simulink model "control"  (R2017b)
settings: Solver=ode45  StartTime=0.0  StopTime=2  RelTol=1e-3
values from neighbouring files (symbols this model uses):
  duracion = in(9)    [GTCL_R3GDL.m]
  Kd = [1.3735e+01 2.5872e+01 0.2837e+01]    [Control.m]    (also in dsgn_PD.m = Kp.*Td)
  Ki = [0 0 0]    [Control.m]    (also in dsgn_PD.m = Kp./Ti)
  Kp = [7.4989e+02 1.4125e+03 1.5488e+02]    [Control.m]    (also in dsgn_PD.m = [2.1312e+06 8.4844e+05 4.5042e+05])
  n = in(7)    [GTCL_R3GDL.m]
  XYZfin = [in(4) in(5) in(6)]'    [GTCL_R3GDL.m]
undefined symbols (not defined in the file or in its folder): t_ini, XYZini
settings Model: Creator=fevaf  LastModifiedBy=Raúl

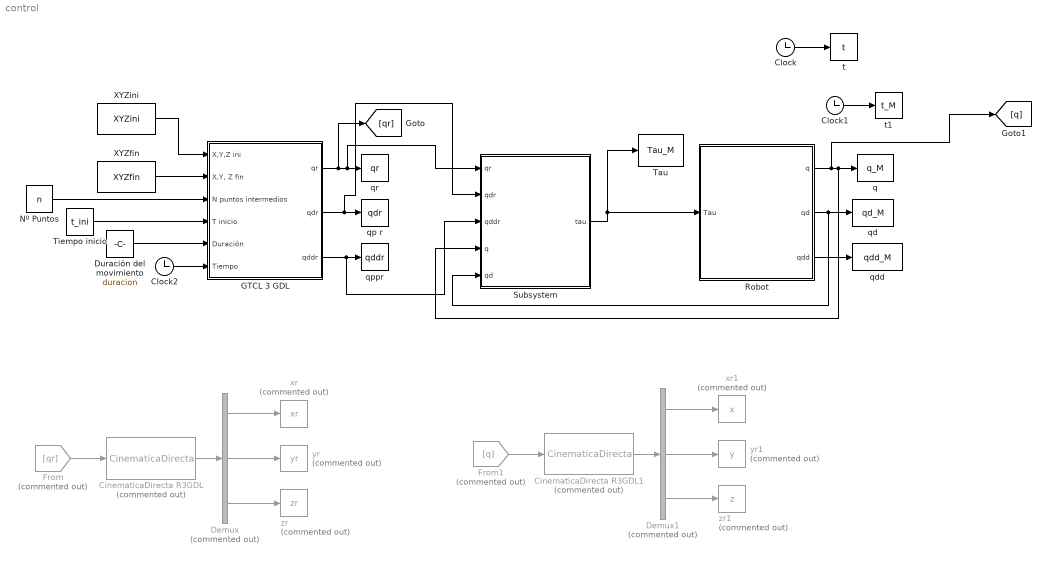
== system control ==
  CinematicaDirecta R3GDL : MATLABFcn  Commented=on  MATLABFcn=CinematicaDirecta
  CinematicaDirecta R3GDL1 : MATLABFcn  Commented=on  MATLABFcn=CinematicaDirecta
  Clock : Clock
  Clock1 : Clock
  Clock2 : Clock
  Demux : Demux  Commented=on  Outputs=3
  Demux1 : Demux  Commented=on  Outputs=3
  Duración del movimiento : Constant  Value=duracion
  From : From  Commented=on  GotoTag=qr
      settings: CloseFcn=tagdialog Close
  From1 : From  Commented=on  GotoTag=q
      settings: CloseFcn=tagdialog Close
  GTCL 3 GDL : Subsystem
  Nº Puntos : Constant  Value=n
  Robot : Subsystem
  Subsystem : Subsystem
  "Tau " : ToWorkspace  VariableName=Tau_M  SampleTime=-1
  Tiempo inicio : Constant  Value=t_ini
  XYZfin : Constant  Value=XYZfin
  XYZini : Constant  Value=XYZini
  q : ToWorkspace  VariableName=q_M  SampleTime=-1
  qd : ToWorkspace  VariableName=qd_M  SampleTime=-1
  qdd : ToWorkspace  VariableName=qdd_M  SampleTime=-1
  qp r : ToWorkspace  VariableName=qdr  SampleTime=-1
  qppr : ToWorkspace  VariableName=qddr  SampleTime=-1
  qr : ToWorkspace  VariableName=qr  SampleTime=-1
  t : ToWorkspace  VariableName=t  SampleTime=-1
  t1 : ToWorkspace  VariableName=t_M  SampleTime=-1
  xr : ToWorkspace  Commented=on  VariableName=xr  SampleTime=-1
  xr1 : ToWorkspace  Commented=on  VariableName=x  SampleTime=-1
  yr : ToWorkspace  Commented=on  VariableName=yr  SampleTime=-1
  yr1 : ToWorkspace  Commented=on  VariableName=y  SampleTime=-1
  zr : ToWorkspace  Commented=on  VariableName=zr  SampleTime=-1
  zr1 : ToWorkspace  Commented=on  VariableName=z  SampleTime=-1
  wires:
  Demux/3 -> zr/1
  Demux/1 -> xr/1
  Demux/2 -> yr/1
  XYZfin/1 -> GTCL 3 GDL/2("X,Y, Z fin")
  XYZini/1 -> GTCL 3 GDL/1(X,Y,Z ini)
  Tiempo inicio/1 -> GTCL 3 GDL/4(T inicio)
  GTCL 3 GDL/3(qddr) -> Subsystem/3(qddr), qppr/1
  CinematicaDirecta R3GDL/1 -> Demux/1
  GTCL 3 GDL/1(qr) -> Subsystem/1(qr), qr/1, [qr]
  Clock2/1 -> GTCL 3 GDL/6(Tiempo)
  Duración del movimiento/1 -> GTCL 3 GDL/5(Duración)
  From/1 -> CinematicaDirecta R3GDL/1
  GTCL 3 GDL/2(qdr) -> Subsystem/2(qdr), qp r/1
  Nº Puntos/1 -> GTCL 3 GDL/3(N puntos intermedios)
  Clock/1 -> t/1
  Subsystem/1("tau ") -> Robot/1(Tau), "Tau "/1
  Robot/2(qd) -> Subsystem/5(qd), qd/1
  Robot/1(q) -> [q], Subsystem/4(q), q/1
  Robot/3(qdd) -> qdd/1
  Clock1/1 -> t1/1
  From1/1 -> CinematicaDirecta R3GDL1/1
  Demux1/2 -> yr1/1
  CinematicaDirecta R3GDL1/1 -> Demux1/1
  Demux1/3 -> zr1/1
  Demux1/1 -> xr1/1

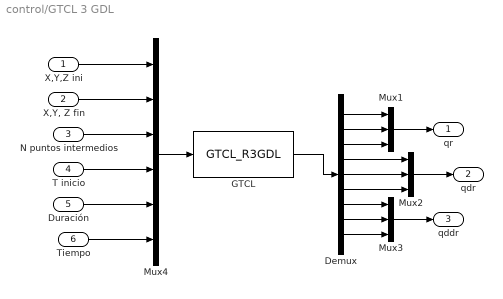
== system control/GTCL 3 GDL ==
  X,Y,Z ini : Inport
  "X,Y, Z fin" : Inport  Port=2
  N puntos intermedios : Inport  Port=3
  T inicio : Inport  Port=4
  Duración : Inport  Port=5
  Tiempo : Inport  Port=6
  Demux : Demux  Outputs=9
  GTCL : MATLABFcn  MATLABFcn=GTCL_R3GDL  OutputDimensions=9
  Mux1 : Mux  Inputs=3
  Mux2 : Mux  Inputs=3
  Mux3 : Mux  Inputs=3
  Mux4 : Mux  Inputs=6
  qr : Outport
  qdr : Outport  Port=2
  qddr : Outport  Port=3
  wires:
  Mux1/1 -> qr/1
  Mux4/1 -> GTCL/1
  X,Y,Z ini/1 -> Mux4/1
  "X,Y, Z fin"/1 -> Mux4/2
  N puntos intermedios/1 -> Mux4/3
  T inicio/1 -> Mux4/4
  Duración/1 -> Mux4/5
  Tiempo/1 -> Mux4/6
  GTCL/1 -> Demux/1
  Demux/1 -> Mux1/1
  Demux/2 -> Mux1/2
  Demux/3 -> Mux1/3
  Mux2/1 -> qdr/1
  Demux/4 -> Mux2/1
  Demux/5 -> Mux2/2
  Demux/6 -> Mux2/3
  Mux3/1 -> qddr/1
  Demux/7 -> Mux3/1
  Demux/8 -> Mux3/2
  Demux/9 -> Mux3/3

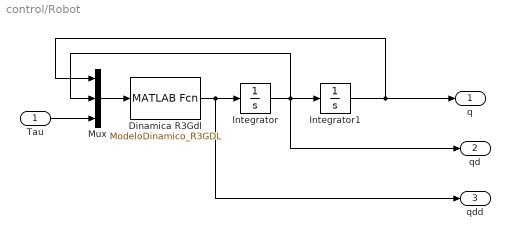
== system control/Robot ==
  Tau : Inport
  Dinamica R3Gdl : MATLABFcn  MATLABFcn=ModeloDinamico_R3GDL
  Integrator : Integrator  InitialCondition=[0;0;0];
  Integrator1 : Integrator  InitialCondition=[0;0;0]
  Mux : Mux  Inputs=3
  q : Outport
  qd : Outport  Port=2
  qdd : Outport  Port=3
  wires:
  Mux/1 -> Dinamica R3Gdl/1
  Dinamica R3Gdl/1 -> Integrator/1, qdd/1
  Integrator/1 -> Integrator1/1, qd/1, Mux/2
  Integrator1/1 -> q/1, Mux/1
  Tau/1 -> Mux/3

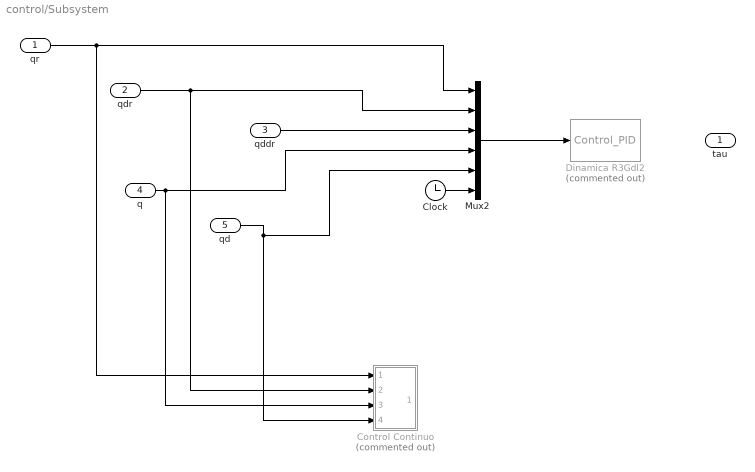
== system control/Subsystem ==
  qr : Inport
  qdr : Inport  Port=2
  qddr : Inport  Port=3
  q : Inport  Port=4
  qd : Inport  Port=5
  Clock : Clock
  "Control Continuo " : Subsystem  Commented=on
  Dinamica R3Gdl2 : MATLABFcn  Commented=on  MATLABFcn=Control_PID  SampleTime=1e-3
  Mux2 : Mux  Inputs=6
  "tau " : Outport
  wires:
  Mux2/1 -> Dinamica R3Gdl2/1
  qr/1 -> "Control Continuo "/1(In1), Mux2/1
  qdr/1 -> "Control Continuo "/2(In2), Mux2/2
  qddr/1 -> Mux2/3
  q/1 -> "Control Continuo "/3(In3), Mux2/4
  qd/1 -> "Control Continuo "/4(In4), Mux2/5
  Clock/1 -> Mux2/6

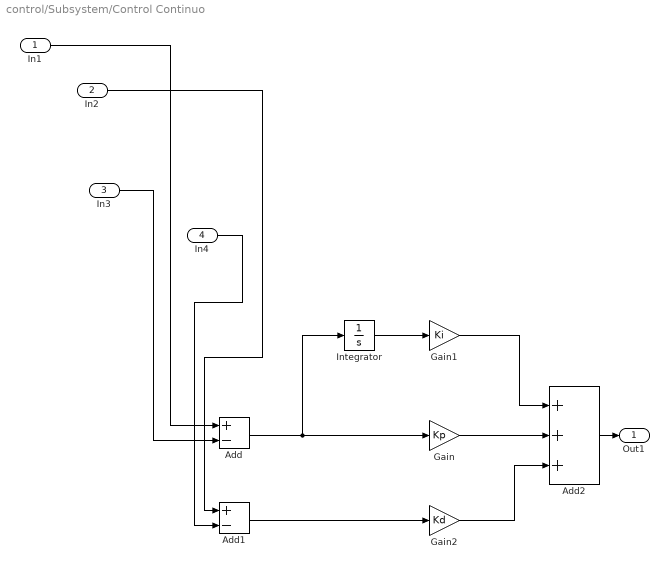
== system control/Subsystem/Control Continuo  ==
  In1 : Inport
  In2 : Inport  Port=2
  In3 : Inport  Port=3
  In4 : Inport  Port=4
  Add : Sum  Inputs=+-
  Add1 : Sum  Inputs=+-
  Add2 : Sum  Inputs=+++
  Gain : Gain  Gain=Kp
  Gain1 : Gain  Gain=Ki
  Gain2 : Gain  Gain=Kd
  Integrator : Integrator
  Out1 : Outport
  wires:
  Add/1 -> Gain/1, Integrator/1
  Integrator/1 -> Gain1/1
  Gain2/1 -> Add2/3
  Add1/1 -> Gain2/1
  Gain/1 -> Add2/2
  Gain1/1 -> Add2/1
  In2/1 -> Add1/1
  In4/1 -> Add1/2
  In1/1 -> Add/1
  Add2/1 -> Out1/1
  In3/1 -> Add/2
